simulink library "init"  (R2024a)
settings: Solver=VariableStepAuto  StartTime=0.0  StopTime=10.0  RelTol=1e-3
settings Model: Creator=adriaeik  LastModifiedBy=adriaeik

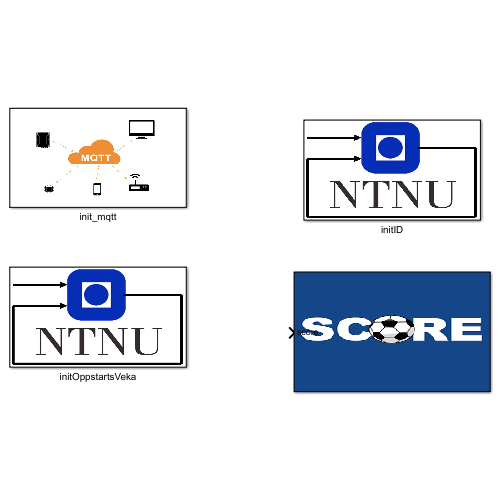
[thumbnail: Simulink's stored preview of the top-level diagram]
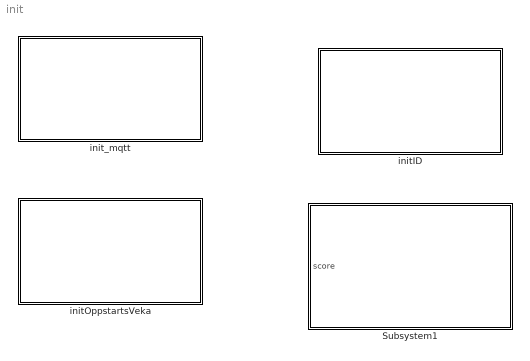
== system init ==
  Subsystem1 : Subsystem
      mask Display: image('score.png');
  initID : Subsystem  mask{carID=0, groupID=0}
      mask prompts: carID "Zumo Car ID"; groupID "Group ID"
      mask Display: image('kyb.png');
  initOppstartsVeka : Subsystem  mask{carID=14, groupID=14}
      mask prompts: carID "Zumo Car ID"; groupID "Group ID"
      mask Display: image('pic/kyb.png');
  init_mqtt : Subsystem  mask{carID=14, groupID=14, brokerVal='192.168.1.3', portVal='1883', userVal='BIAISbroker', passVal='shinyteapot294'}
      mask prompts: carID "Zumo Car ID"; groupID "Group ID"; brokerVal "Broker"; portVal "MQTT-port"; userVal "Username"; passVal "Password"
      mask Display: image('pic/mqtt.png');

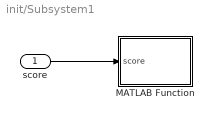
== system init/Subsystem1 ==
  score : Inport
  MATLAB Function : MATLAB Function  TreatAsAtomicUnit=on
  wires:
  score/1 -> MATLAB Function/1(score)

== system init/initID ==

== system init/initOppstartsVeka ==

== system init/init_mqtt ==

== matlab function init/Subsystem1/MATLAB Function ==
  data: score input
function fcn(score)
 assignin('base', 'score', score);
